simulink subsystem "joystick_controller"  (R2025b)
settings: Solver=VariableStepAuto  StartTime=0.0  StopTime=10.0  RelTol=1e-3
libraries: ros2lib x1
settings Model: Creator=kjhaydon  LastModifiedBy=vulcangrip

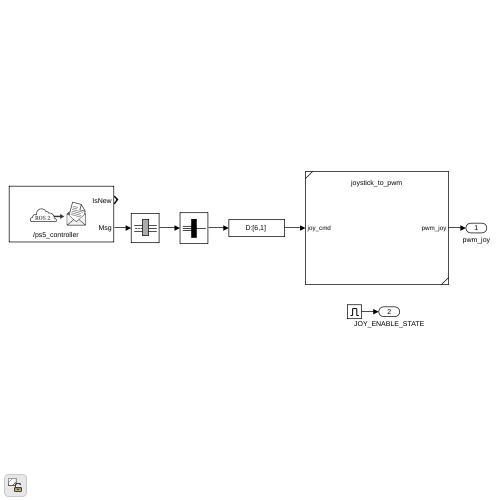
[thumbnail: Simulink's stored preview of the top-level diagram]
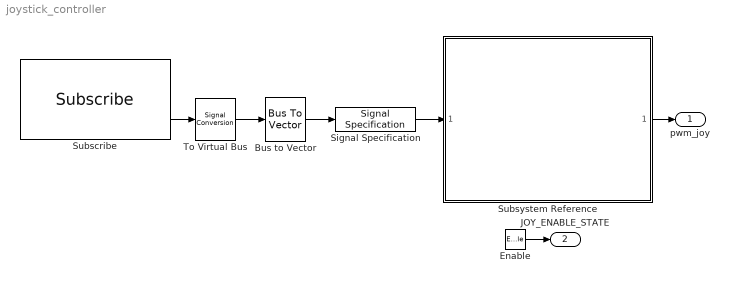
== system joystick_controller ==
  Enable : EnablePort  ShowOutputPort=on
  Bus to Vector : BusToVector
  Signal Specification : SignalSpecification  Dimensions=[6,1]
  Subscribe : ros2lib/Subscribe  topicSource=Specify your own  topic=/ps5_controller  messageType=remote_control_interface/Gamepad  sampleTime=1/60  QOSHistory=Keep last  QOSDepth=10  QOSReliability=Reliable  QOSDurability=Volatile  QOSDeadline=Inf  QOSLifespan=Inf  QOSLiveliness=Automatic  QOSLeaseDuration=Inf  QOSAvoidROSNamespaceConventions=off
  Subsystem Reference : Subsystem  ReferencedSubsystem=joystick_to_pwm
  To Virtual Bus : SignalConversion  OverrideOpt=off
  pwm_joy : Outport
  JOY_ENABLE_STATE : Outport  Port=2
  wires:
  Signal Specification/1 -> Subsystem Reference/1
  Subscribe/2 -> To Virtual Bus/1
  Bus to Vector/1 -> Signal Specification/1
  To Virtual Bus/1 -> Bus to Vector/1
  Enable/1 -> JOY_ENABLE_STATE/1
  Subsystem Reference/1 -> pwm_joy/1
